simulink library "Simple_lib"  (R2018b)
settings: Solver=ode45  StartTime=0.0  StopTime=10.0  RelTol=1e-3  EnableMultiTasking=on
undefined symbols (not defined in the file or in its folder): Acceptance, beta, C, C_J, C_P, c_wall, dGain, DiscIntNeverNeededParam, Duplex, Electrical_lib, grab, h_fe, i, i3, K_T, Kman, KmanCE, mu_s, n_rev, R_arm, Simplex, systemTs, tau_0, TinIC, Ts, w_0, wallMass, Watch_lib
libraries: $bdroot x407, PlantUtilityBlockset_lib x30, peGeneralControl x22, simulink x11
(part 1 of 14)
settings Model: Creator=Bill Weston  LastModifiedBy=billw
settings DataIOCC: LimitDataPoints=on  SaveFormat=Array  SignalLoggingSaveFormat=ModelDataLogs
settings OptimizationCC: ExpressionDepthLimit=2147483647  LifeSpan=inf
settings DebuggingCC: UnderspecifiedInitializationDetection=Classic  MergeDetectMultiDrivingBlocksExec=none  SolverPrmCheckMsg=warning  FcnCallInpInsideContextMsg=warning  StateNameClashWarn=warning  SFUnexpectedBacktrackingDiag=warning  SFNoUnconditionalDefaultTransitionDiag=warning  SFExecutionAtInitializationDiag=none
settings HardwareCC: ProdBitPerPointer=32  ProdBitPerSizeT=32  ProdBitPerPtrDiffT=32  ProdLargestAtomicFloat=None  ProdIntDivRoundTo=Undefined  ProdEndianess=Unspecified  ProdWordSize=32  ProdHWDeviceType=32-bit Generic
settings ModelReferenceCC: PropagateSignalLabelsOutOfModel=off
settings SFSimCC: SimUseLocalCustomCode=off
settings RTWCC: RTWUseLocalCustomCode=off
settings CodeAppCC: StateflowObjectComments=on
settings GRTTargetCC: TargetLangStandard=C89/C90 (ANSI)  GeneratePreprocessorConditionals=Disable all  CombineOutputUpdateFcns=off  GRTInterface=on
settings ConfigComp: CovMetricSettings=dw  CovHtmlReporting=on  CovSaveCumulativeToWorkspaceVar=on  CovSaveSingleToWorkspaceVar=on  CovExternalEMLEnable=off

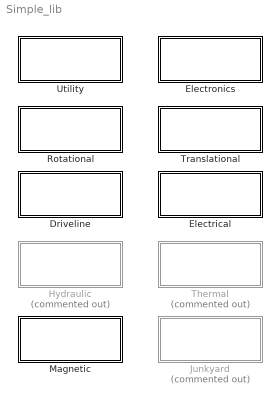
== system Simple_lib ==
  Driveline : Subsystem
  Electrical : Subsystem
  Electronics : Subsystem
  Hydraulic : Subsystem  Commented=on
  Junkyard : Subsystem  Commented=on
  Magnetic : Subsystem
  Rotational : Subsystem
  Thermal : Subsystem  Commented=on
  Translational : Subsystem
  Utility : Subsystem

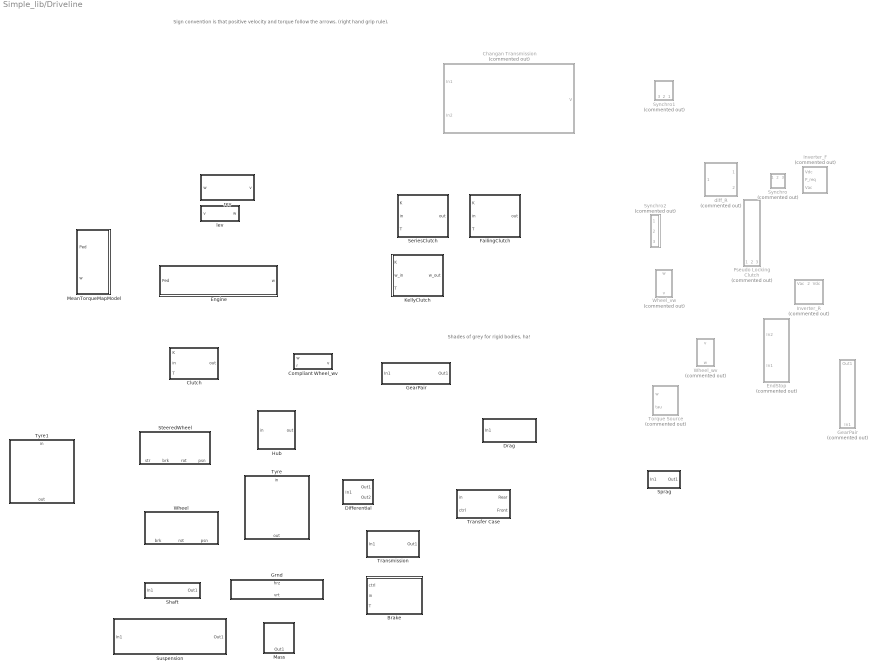
== system Simple_lib/Driveline ==
  note: Shades of grey for rigid bodies, ha!
  note: Sign convention is that positive velocity and torque follow the arrows. (right hand grip rule).
  Brake : Subsystem
      mask Display:
      | %plot([0.2 0 0.8 0.9 1 0.9 0.8 0 0.2],[0 0.9 1 0.8 0 -0.8 -1 -0.9 0])
      | 
      | plot([1 1],[1 -1]*0.75)
      | plot([0 0.8],[0 0]*0.75)
      | 
      | color('orange')
      | plot([1 0],[-1 -1]*0.75)
      | color('black')
      | plot([0 1],[1 1]*0.75)
      | 
      | 
      | 
      | color('white')
      | plot([0 1.01], [1.1 1.1])
      | plot([0 1.01], [-1.1 -1.1])
  Changan Transmission : Subsystem  Commented=on
      mask Display:
      | %image('C:\Projects\Descartes__confidential__\model\Transmission_DCT400H.png');
      | plot([0 1 1 0 0],[1 0.7 -0.7 -1 1])
      | 
      | color('white')
      | plot([0 1.01], [1.1 1.1])
      | plot([0 1.01], [-1.1 -1.1])
  Clutch : Subsystem  mask{w_0=0, grab=.1, I=0}
      mask prompts: w_0 "Initial output speed (rad/s)"; grab "Sharpness of clutch grab (-)"; I "Inertia at output (kgm^2)"
      mask Display:
      | %color('gray')
      | %plot([-1 1 1 -1 -1], [-1 -1 1 1 -1])
      | %color('black')
      | %plot([1.0 1.18 1.18 1.0], [0 .2 -.2 0])
      | 
      | plot([-10 -5],[0 0]);
      | plot([5 10],[0 0]);
      | 
      | patch(-[3 3 5 5],[-1  1 1 -1]*(50+50));
      | patch([3 3 5 5],[-1  1 1 -1]*(50+50));
  Compliant Wheel_wv : Subsystem
      mask Display:
      | %color('white');
      | %plot([0 0],[-1 1]);
      | %plot([1 1],[-1 -1]);
      | %color('black')
      | plot([0 1],[1 1]/2.5);
      | plot([1 1],[-1  1]);
  Differential : Subsystem  mask{r=.2}
      mask prompts: r "Ratio (speed_out/speed_in)"
      mask Display:
      | plot([0 1 1 0 0],[0.7 1 -1 -0.7 0.7])
      | 
      | color('white')
      | plot([0 1.01], [1.1 1.1])
      | plot([0 1.01], [-1.1 -1.1])
  Drag : Subsystem
  EndStop : Subsystem  Commented=on  mask{k=10000}
      mask prompts: k "Stiffness (N/rad)"
      mask Display:
      | %color('black')
      | plot(   [    0     0.3827     0.7071     0.9239     1.0000     0.9239     0.7071     0.3827     0.0000    -0.3827    -0.7071    -0.9239    -1.0000    -0.9239    -0.7071    -0.3827    -0.0000     0.3827     0.7071     0.9239     1.0000     0.9239     0.7071     0.3827     0.0000    -0.3827    -0.7071    -0.9239    -1.0000    -0.9239    -0.7071    -0.3827    -0.0000     0.3827     0.7071     0.9239     1.0000     0.9239     0.7071     0.3827     0.0000    -0.3827    -0.7071    -0.9239    -1.0000    -0.9239    -0.7071    -0.3827    -0.0000     0.3827     0.7071     0.9239     1.0000     0.9239     0.7071     0.3827     0.0000    -0.3827    -0.7071    -0.9239    -1.0000    -0.9239    -0.7071    -0.3827    -0.0000],   -1.25+.5*[-0.0625    -0.0421    -0.0129     0.0230     0.0625     0.1020     0.1379     0.1671     0.1875     0.1984     0.2004     0.1958     0.1875     0.1792     0.1746     0.1766     0.1875     0.2079     0.2371     0.2730     0.3125     0.3520     0.3879     0.4171     0.4375     0.4484     0.4504     0.4458     0.4375     0.4292     0.4246     0.4266     0.4375     0.4579     0.4871     0.5230     0.5625     0.6020     0.6379     0.6671     0.6875     0.6984     0.7004     0.6958     0.6875     0.6792     0.6746     0.6766     0.6875     0.7079     0.7371     0.7730     0.8125     0.8520     0.8879     0.9171     0.9375     0.9484     0.9504     0.9458     0.9375     0.9292     0.9246     0.9266     0.9375])
      | plot(   [    0     0.3827     0.7071     0.9239     1.0000     0.9239     0.7071     0.3827     0.0000    -0.3827    -0.7071    -0.9239    -1.0000    -0.9239    -0.7071    -0.3827    -0.0000     0.3827     0.7071     0.9239     1.0000     0.9239     0.7071     0.3827     0.0000    -0.3827    -0.7071    -0.9239    -1.0000    -0.9239    -0.7071    -0.3827    -0.0000     0.3827     0.7071     0.9239     1.0000     0.9239     0.7071     0.3827     0.0000    -0.3827    -0.7071    -0.9239    -1.0000    -0.9239    -0.7071    -0.3827    -0.0000     0.3827     0.7071     0.9239     1.0000     0.9239     0.7071     0.3827     0.0000    -0.3827    -0.7071    -0.9239    -1.0000    -0.9239    -0.7071    -0.3827    -0.0000],   1.25+.5*[-0.0625    -0.0421    -0.0129     0.0230     0.0625     0.1020     0.1379     0.1671     0.1875     0.1984     0.2004     0.1958     0.1875     0.1792     0.1746     0.1766     0.1875     0.2079     0.2371     0.2730     0.3125     0.3520     0.3879     0.4171     0.4375     0.4484     0.4504     0.4458     0.4375     0.4292     0.4246     0.4266     0.4375     0.4579     0.4871     0.5230     0.5625     0.6020     0.6379     0.6671     0.6875     0.6984     0.7004     0.6958     0.6875     0.6792     0.6746     0.6766     0.6875     0.7079     0.7371     0.7730     0.8125     0.8520     0.8879     0.9171     0.9375     0.9484     0.9504     0.9458     0.9375     0.9292     0.9246     0.9266     0.9375])
      | color('white')
      | plot([-1 1 1 -1 -1], [-1 -1 1 1 -1])
  Engine : Subsystem  mask{w_0=0, I=.2}
      mask prompts: w_0 "Initial speed (rad/s)"; I "Inertia"
      mask Display:
      | %color('white');
      | %plot([-4.4 4.4],[1 1]);
      | %plot([-4.4 4.4],[-1 -1]);
      | %color('black')
      | 
      | plot(-3.3+[-1 -.9 -.5 0 .5 .9 1  .9  .5  0 -.5 -.9 -1],      [ 0  .5 .9 1 .9 .5 0 -.5 -.9 -1 -.9 -.5  0]);
      | plot(-1.1+[-1 -.9 -.5 0 .5 .9 1  .9  .5  0 -.5 -.9 -1],      [ 0  .5 .9 1 .9 .5 0 -.5 -.9 -1 -.9 -.5  0]);
      | plot(1.1+[-1 -.9 -.5 0 .5 .9 1  .9  .5  0 -.5 -.9 -1],      [ 0  .5 .9 1 .9 .5 0 -.5 -.9 -1 -.9 -.5  0]);
      | plot(3.3+[-1 -.9 -.5 0 .5 .9 1  .9  .5  0 -.5 -.9 -1],      [ 0  .5 .9 1 .9 .5 0 -.5 -.9 -1 -.9 -.5  0]);
      | 
      | patch([4.8 5 5 4.8], [-1 -1 1 1])
      | plot([4.3 5], [0 0])
  FailingClutch : Subsystem  mask{w_0=0}
      mask prompts: w_0 "Initial speed (rad/s)"
      mask Display:
      | %color('gray')
      | plot([-1 1 1 -1 -1], [-1 -1 1 1 -1])
      | %color('black')
      | %plot([1.0 1.18 1.18 1.0], [0 .2 -.2 0])
  GearPair : Subsystem  mask{n_i=19, n_o=23}
      mask prompts: n_i "Number of input teeth"; n_o "Number of output teeth"
      mask Display:
      | plot([-n_i -5],[0 0]);
      | plot([5 n_o],[0 0]);
      | 
      | patch(-[3 3 5 5],[-1  1 1 -1]*(n_i+n_o));
      | patch([3 3 5 5],[-1  1 1 -1]*(n_i+n_o));
  "GearPair " : Subsystem  Commented=on  mask{n_i=75, n_o=16}
      mask prompts: n_i "Number of input teeth"; n_o "Number of output teeth"
      mask Display:
      | %plot([-n_i -5],[0 0]);
      | %plot([5 n_o],[0 0]);
      | 
      | patch(-[5 5 n_i n_i],[-1  1 1 -1]*(n_i+n_o),[1 1 1]*.8);
      | patch([5 5 n_o n_o],[-1  1 1 -1]*(n_i+n_o),[1 1 1]*.8);
      | 
      | color('black')
      | plot([-n_i -3],[1 1]*(n_i+n_o));
      | plot([3 n_o],[1 1]*(n_i+n_o));
      | 
      | plot([-n_i -3],-[1 1]*(n_i+n_o));
      | plot([3 n_o],-[1 1]*(n_i+n_o));
      | 
      | 
      | patch(-[3 3 5 5],[-1  1 1 -1]*(n_i+n_o),[0 0 0]);
      | patch([3 3 5 5],[-1  1 1 -1]*(n_i+n_o),[0 0 0]);
  Grnd : Subsystem
      mask Display:
      | %color('white')
      | %plot([-1 1 1 -1 -1], [-1 -1 1 1 -1])
      | 
      | %color('black')
      | %plot([1.0 1.18 1.18 1.0], [0 .15 -.15 0])
      | 
      | %color('green')
      | plot([0.3 0.4 0.39 0.42 0.39 0.4 0.405 0.41 0.39 0.39 0.41],[-1 -.8 -.6 -.4 -.2 0 .2 .4 .6 .8 1])
      | plot([1.0 0.4], [-1.0 -0.6])
      | %color('yellow')
      | plot([1.0 0.4], [-0.7 -0.3])
      | %color('green')
      | plot([1.0 0.4], [-0.4 0.0])
      | %color('yellow')
      | plot([1.0 0.4], [-0.1 0.3])
      | %color('green')
      | plot([1.0 0.4], [0.2 0.6])
      | %color('yellow')
      | plot([1.0 0.4], [0.5 0.9])
      | 
      | %plot([-0.4 1],[0 0])
  Hub : Subsystem  mask{I=1}
      mask prompts: I "Inertia (kgm^2)"
      mask Display:
      | %color('white');
      | %plot([0 4],[1 1]);
      | %plot([0 4],[-1 -1]);
      | %color('black')
      | %plot([0 2],[0 0]);
      | plot([-1 -.9 -.5 0 .5 .9 1  .9  .5  0 -.5 -.9 -1],     [ 0  .5 .9 1 .9 .5 0 -.5 -.9 -1 -.9 -.5  0]);
      | plot([-1 -.9 -.5 0 .5 .9 1  .9  .5  0 -.5 -.9 -1]*.25,      [ 0  .5 .9 1 .9 .5 0 -.5 -.9 -1 -.9 -.5  0]*.25);
      | patch([-1 1 1 -1]*.1  +.5,[1 1 -1 -1]*.1+.4)
      | patch([-1 1 1 -1]*.1  +.5,[1 1 -1 -1]*.1-.4)
      | patch([-1 1 1 -1]*.1  -.2,[1 1 -1 -1]*.1+.6)
      | patch([-1 1 1 -1]*.1  -.2,[1 1 -1 -1]*.1-.6)
      | patch([-1 1 1 -1]*.1  -.6,[1 1 -1 -1]*.1+0)
  Inverter_F : Subsystem  Commented=on
  Inverter_R : Subsystem  Commented=on
  KellyClutch : Subsystem  mask{w_drop=0}
      mask prompts: w_drop "Speed drop (rads per sec)"
      mask Display:
      | %color('gray')
      | plot([-1 1 1 -1 -1], [-1 -1 1 1 -1])
      | %color('black')
      | %plot([1.0 1.18 1.18 1.0], [0 .2 -.2 0])
  Mass : Subsystem  mask{I=10000, v_0=[0 0 0]'}
      mask prompts: I "Inertia (kg)"; v_0 "Initial speed of inertia [3] (m/s)"
      mask Display:
      | plot([0 1 1 0 0],[1 1 -1 -1 1])
      | 
      | color('white')
      | plot([0 1.01], [1.1 1.1])
      | plot([0 1.01], [-1.1 -1.1])
  MeanTorqueMapModel : Subsystem
      mask Display:
      | plot( [-.7 0],[-1.1 0.3] )
      | plot( .9*[-1 -.8 .8 1 ],.3*[ .6 1 1 .6] )
      | 
      | color('black')
      | plot( [1 1 -1 -1],[0 1 1 0] )
      | plot( [1 1 -1 -1]*0.9,[0.95 1 1 0.95]*1.1 )
      | plot( [1 1 -1 -1]*0.81,[0.95 1 1 0.95]*1.2 )
      | plot( [1 1 -1 -1]*0.72,[0.95 1 1 0.95]*1.3 )
      | color('white')
      | %plot([-1 1], [1.1 1.1])
      | plot([-1 1 1 -1 -1]*1.1, -[-1 -1 1 1 -1]*2)
  Pseudo Locking Clutch : Subsystem  Commented=on
      mask Display:
      | patch([0 1 1 0],[1 1 .9 .9]);
      | patch([0 1 1 0],-[1 1 .9 .9]);
  SeriesClutch : Subsystem  mask{w_drop=0}
      mask prompts: w_drop "Speed drop (rads per sec)"
      mask Display:
      | %color('gray')
      | plot([-1 1 1 -1 -1], [-1 -1 1 1 -1])
      | %color('black')
      | %plot([1.0 1.18 1.18 1.0], [0 .2 -.2 0])
  Shaft : Subsystem  mask{k=10, b=.1, I=.2, w_0=0}
      mask prompts: k "Stiffness (Nm/rad)"; b "Damping (Nms/rad)"; I "Inertia (kgm^2)"; w_0 "Initial speed of inertia (rad/s)"
      mask Display:
      | plot([0 1 1 0 0],[1 1 -1 -1 1])
      | 
      | color('white')
      | plot([0 1.01], [1.1 1.1])
      | plot([0 1.01], [-1.1 -1.1])
  Sprag : Subsystem  mask{deltaV=0}
      mask prompts: deltaV "Potential Drop (V)"
      mask Display:
      | patch( [1 1.05 1.05 1],[-1 -1 1 1])
      | patch( [1 0 0],[0 1 -1])
  SteeredWheel : Subsystem
      mask Display:
      | plot([-.8 -1 -1 -.8 .8 1 1 .8 -.8], [-1 -.9 .9 1 1 .9 -.9 -1 -1])
      | 
      | plot([.1 .2 .1 .2 .1 .2 .1 .2 .1 .2 .1]-.7, [0 1 2 3 4 5 6 7 8 9 10]*.2-1)
      | plot([.1 .2 .1 .2 .1 .2 .1 .2 .1 .2 .1]-.4, [0 1 2 3 4 5 6 7 8 9 10]*.2-1)
      | plot([.1 .2 .1 .2 .1 .2 .1 .2 .1 .2 .1]-.1, [0 1 2 3 4 5 6 7 8 9 10]*.2-1)
      | plot([.1 .2 .1 .2 .1 .2 .1 .2 .1 .2 .1]+.2, [0 1 2 3 4 5 6 7 8 9 10]*.2-1)
      | plot([.1 .2 .1 .2 .1 .2 .1 .2 .1 .2 .1]+.5, [0 1 2 3 4 5 6 7 8 9 10]*.2-1)
      | 
      | patch([-1 -1 -1.6 -1.6], [-0.1 0.01 0.01 -0.1])
      | plot([-1.4 -1.4],[0.4 -0.4])
      | 
      | color('cyan') % steering
      | plot([-1.6 -1.1],[1.2 .6])
      | 
      | color('gray') % suspension
      | plot([-1 -.9 -.5 0 .5 .9 1  .9  .5  0 -.5 -.9 -1]*.7-.8,      [ 0  .5 .9 1 .9 .5 0 -.5 -.9 -1 -.9 -.5  0]*.2-.8);
      | plot([-1 -.9 -.5 0 .5 .9 1  .9  .5  0 -.5 -.9 -1]*.7-.8,      [ 0  .5 .9 1 .9 .5 0 -.5 -.9 -1 -.9 -.5  0]*.2-.7);
      | plot([-1 -.9 -.5 0 .5 .9 1  .9  .5  0 -.5 -.9 -1]*.7-.8,      [ 0  .5 .9 1 .9 .5 0 -.5 -.9 -1 -.9 -.5  0]*.2-.6);
      | plot([-1 -.9 -.5 0 .5 .9 1  .9  .5  0 -.5 -.9 -1]*.5-.8,      [ 0  .5 .9 1 .9 .5 0 -.5 -.9 -1 -.9 -.5  0]*.15-.5);
      | patch([-1 -1 -.8 -.8],[0 -0.7 -0.7 0],[1 1 1]*.5)
      | 
      | color('black') % brakes
      | plot([-1.2 -1.2 -1.6 -1.6],[0.2 0.6 0.6 0.2])
      | 
      | color('white')
      | plot([-1.6 1.1], [-1.1 -1.1])
      | plot([-1.6 1.1], [1.6 1.6])
  Suspension : Subsystem  mask{k=1e5, b=100, I=10, v_0=0}
      mask prompts: k "Stiffness (N)"; b "Damping (Ns)"; I "Inertia (kg)"; v_0 "Initial speed of inertia (m/s)"
      mask Display:
      | plot([0 1 1 0 0],[1 1 -1 -1 1])
      | plot([0 -1 -1 0 0],[1 1 -1 -1 1]*.7)
      | plot([-1 -.9 -.7 -.5 -.3 -.1 0],[0 1 -1 1 -1 1 0])
      | color('white')
      | plot([0 1.01], [1.1 1.1])
      | plot([0 1.01], [-1.1 -1.1])
  Synchro : Subsystem  Commented=on
      mask Display:
      | %patch([-1 0 0 -1], [1 .9 1 .9]);
      | patch([1 1 0.4 -0.4 -1 -1], [1 .6 -.2 -.2 .6 1],[1 0 0]);
      | patch([1 1 0.4 -0.4 -1 -1], -[1 0 .8 .8 0 1], [0 0 0]);
      | %color('white');
      | %plot([-1 -1],[-1 1]);
      | %plot([1 1],[-1 1]);
  Synchro1 : Subsystem  Commented=on
      mask Display:
      | %color('black')
      | %patch([-1 0 0 -1], [1 .9 1 .9]);
      | patch([1 1 0.4 -0.4 -1 -1], [1 .6 -.2 -.2 .6 1]);
      | patch([1 1 0.4 -0.4 -1 -1], -[1 0 .8 .8 0 1]);
      | color('white');
      | plot([-1 -1],[-1 1]);
      | plot([1 1],[-1 1]);
  Synchro2 : Subsystem  Commented=on  InitFcn=bond
      mask Display:
      | color('white');
      | plot([0 1],[3 3]);
      | plot([0 1],[-3 -3]);
      | color('black')
      | plot([0 1],[0 2]);
      | plot([0 1],[-2 -0]);
  Torque Source : Subsystem  Commented=on
      mask Display:
      | plot([ 1 0 -.5 -.9 -1 -.9 -.5  0 1 ], -[ 1 1  .9  .5  0 -.5 -.9 -1 -1]);
      | plot([ 1 1 ], [-1 1]);
      | plot([ .8 -.4 ], [0 0]);
      | plot([ 0 -.5 0], [.5 0 -.5]);
      | plot([ 0 -.7 0], [.7 0 -.7]);
  Transfer Case : Subsystem
      mask Display:
      | plot([0 1 1 0 0],[1 0.9 -0.9 -1 1])
      | 
      | color('white')
      | plot([0 1.01], [1.1 1.1])
      | plot([0 1.01], [-1.1 -1.1])
  Transmission : Subsystem  mask{r=2}
      mask prompts: r "Ratio (torque_out/torque_in)"
      mask Display:
      | plot([0 1 1 0 0],[1 0.7 -0.7 -1 1])
      | 
      | color('white')
      | plot([0 1.01], [1.1 1.1])
      | plot([0 1.01], [-1.1 -1.1])
  Tyre : Subsystem  mask{k_lin=2e5, b_lin=1e4, r_0=0.30, I=0.2}
      mask prompts: k_lin "Linear stiffness (N/m)"; b_lin "Linear damping (Ns/m)"; r_0 "Equilibrium radius (m)"; I "Inertia (kgm^2)"
      mask Display:
      | color('gray')
      | patch([[-1 -.9 -.5 0 .5 .9 .9  .9  .5  0 -.5 -.9 -1 ], [-1 -.9 -.5 0 .5 .9 1  .9  .5  0 -.5 -.9 -1]*.7],      [[ 0  .5 .9 1 .9 .5 0 -.5 -.9 -1 -.9 -.5  0], [ 0  -.5 -.9 -1 -.9 -.5 0 .5 .9 1 .9 .5  0]*.7]);
      | 
      | color('gray')
      | plot([-1 -.9 -.5 0 .5 .9 1  .9  .5  0 -.5 -.9 -1]*.8,      [ 0  .5 .9 1 .9 .5 0 -.5 -.9 -1 -.9 -.5  0]*.8);
      | 
      | color('green')
      | plot([-1 -.9 -.5 0 .5 .9 1  .9  .5  0 -.5 -.9 -1]*.15,      [ 0  .5 .9 1 .9 .5 0 -.5 -.9 -1 -.9 -.5  0]*.15);
      | 
      | patch([-1 1 1 -1]*.08  +.5*.6,[1 1 -1 -1]*.08+.4*.6)
      | patch([-1 1 1 -1]*.08  +.5*.6,[1 1 -1 -1]*.08-.4*.6)
      | patch([-1 1 1 -1]*.08 -.2*.6,[1 1 -1 -1]*.08+.6*.6)
      | patch([-1 1 1 -1]*.08 -.2*.6,[1 1 -1 -1]*.08-.6*.6)
      | patch([-1 1 1 -1]*.08 -.6*.6,[1 1 -1 -1]*.08-.0*.6)
      | 
      | %color('white');
  Tyre1 : Subsystem  mask{I=1}
      mask prompts: I "Inertia (kgm^2)"
      mask Display:
      | color('gray')
      | patch([[-1 -.9 -.5 0 .5 .9 .9  .9  .5  0 -.5 -.9 -1 ], [-1 -.9 -.5 0 .5 .9 1  .9  .5  0 -.5 -.9 -1]*.7],      [[ 0  .5 .9 1 .9 .5 0 -.5 -.9 -1 -.9 -.5  0], [ 0  -.5 -.9 -1 -.9 -.5 0 .5 .9 1 .9 .5  0]*.7]);
      | 
      | color('gray')
      | plot([-1 -.9 -.5 0 .5 .9 1  .9  .5  0 -.5 -.9 -1]*.8,      [ 0  .5 .9 1 .9 .5 0 -.5 -.9 -1 -.9 -.5  0]*.8);
      | 
      | color('green')
      | plot([-1 -.9 -.5 0 .5 .9 1  .9  .5  0 -.5 -.9 -1]*.15,      [ 0  .5 .9 1 .9 .5 0 -.5 -.9 -1 -.9 -.5  0]*.15);
      | 
      | patch([-1 1 1 -1]*.08  +.5*.6,[1 1 -1 -1]*.08+.4*.6)
      | patch([-1 1 1 -1]*.08  +.5*.6,[1 1 -1 -1]*.08-.4*.6)
      | patch([-1 1 1 -1]*.08 -.2*.6,[1 1 -1 -1]*.08+.6*.6)
      | patch([-1 1 1 -1]*.08 -.2*.6,[1 1 -1 -1]*.08-.6*.6)
      | patch([-1 1 1 -1]*.08 -.6*.6,[1 1 -1 -1]*.08-.0*.6)
      | 
      | %color('white');
  Wheel : Subsystem
      mask Display:
      | plot([-.8 -1 -1 -.8 .8 1 1 .8 -.8], [-1 -.9 .9 1 1 .9 -.9 -1 -1])
      | 
      | plot([.1 .2 .1 .2 .1 .2 .1 .2 .1 .2 .1]-.7, [0 1 2 3 4 5 6 7 8 9 10]*.2-1)
      | plot([.1 .2 .1 .2 .1 .2 .1 .2 .1 .2 .1]-.4, [0 1 2 3 4 5 6 7 8 9 10]*.2-1)
      | plot([.1 .2 .1 .2 .1 .2 .1 .2 .1 .2 .1]-.1, [0 1 2 3 4 5 6 7 8 9 10]*.2-1)
      | plot([.1 .2 .1 .2 .1 .2 .1 .2 .1 .2 .1]+.2, [0 1 2 3 4 5 6 7 8 9 10]*.2-1)
      | plot([.1 .2 .1 .2 .1 .2 .1 .2 .1 .2 .1]+.5, [0 1 2 3 4 5 6 7 8 9 10]*.2-1)
      | 
      | patch([-1 -1 -1.6 -1.6], [-0.05 0.05 0.05 -0.05])
      | plot([-1.4 -1.4],[0.4 -0.4])
      | 
      | %color('cyan') % steering
      | %plot([-1.6 -1.1],[1.2 .6])
      | 
      | color('gray') % suspension
      | plot([-1 -.9 -.5 0 .5 .9 1  .9  .5  0 -.5 -.9 -1]*.7-.8,      [ 0  .5 .9 1 .9 .5 0 -.5 -.9 -1 -.9 -.5  0]*.2-.8);
      | plot([-1 -.9 -.5 0 .5 .9 1  .9  .5  0 -.5 -.9 -1]*.7-.8,      [ 0  .5 .9 1 .9 .5 0 -.5 -.9 -1 -.9 -.5  0]*.2-.7);
      | plot([-1 -.9 -.5 0 .5 .9 1  .9  .5  0 -.5 -.9 -1]*.7-.8,      [ 0  .5 .9 1 .9 .5 0 -.5 -.9 -1 -.9 -.5  0]*.2-.6);
      | plot([-1 -.9 -.5 0 .5 .9 1  .9  .5  0 -.5 -.9 -1]*.5-.8,      [ 0  .5 .9 1 .9 .5 0 -.5 -.9 -1 -.9 -.5  0]*.15-.5);
      | patch([-1 -1 -.8 -.8],[0 -0.7 -0.7 0],[1 1 1]*.5)
      | 
      | color('black') % brakes
      | plot([-1.2 -1.2 -1.6 -1.6],[0.2 0.6 0.6 0.2])
      | 
      | color('white')
      | plot([-1.1 1.1], [-1.1 -1.1])
      | plot([-1.1 1.1], [1.1 1.1])
  Wheel_vw : Subsystem  Commented=on  InitFcn=bond
      mask Display:
      | %color('white');
      | %plot([0 0],[-1 1]);
      | %plot([1 1],[-1 -1]);
      | %color('black')
      | plot([0 1],[0 0]);
      | plot([0 0],[-1  1]);
  Wheel_wv : Subsystem  Commented=on
      mask Display:
      | %color('white');
      | %plot([0 0],[-1 1]);
      | %plot([1 1],[-1 -1]);
      | %color('black')
      | plot([0 1],[0 0]);
      | plot([1 1],[-1  1]);
  diff_R : Subsystem  Commented=on
  lev : Subsystem  mask{r=1}
      mask prompts: r "Radius (m)"
      settings: AttributesFormatString=%<r>
      mask Display:
      | %color('white');
      | %plot([0 0],[-1 1]);
      | %plot([1 1],[-1 -1]);
      | %color('black')
      | plot([0 1],[1 1]*0);
      | color('darkgreen')
      | plot([0 0],[-1  1]);
  rev : Subsystem  mask{r=n_rev}
      mask prompts: r "Radius (m)"
      settings: AttributesFormatString=%<r>
      mask Display:
      | %color('white');
      | %plot([0 0],[-1 1]);
      | %plot([1 1],[-1 -1]);
      | 
      | 
      | plot([.99 .99],[-1  1]);
      | color('green')
      | plot([0 1],[1 1]*0);
